simulink model "simulate_DSBSC"  (R2021a)
settings: Solver=VariableStepAuto  StartTime=0.0  StopTime=0.1  RelTol=1e-3
InitFcn:
  | fs = 4000;
  | frameSize = 1;
libraries: dspsrcs4 x4, commanapbnd3 x2, dsparch4 x1
settings Model: Creator=Byung-Jun Jang  LastModifiedBy=user
settings SolverCC: AlgebraicLoopSolver=TrustRegion
settings DataIOCC: ReturnWorkspaceOutputs=off
settings DebuggingCC: SFMachineParentedDataDiag=warning  ArithmeticOperatorsInVariantConditions=warning
settings SFSimCC: SimUseLocalCustomCode=off  CustomCodeUndefinedFunction=UseInterfaceOnly
settings RTWCC: RTWUseLocalCustomCode=off
settings CodeAppCC: StateflowObjectComments=on
settings SimscapeCC: SimscapeNormalizeSystem=off

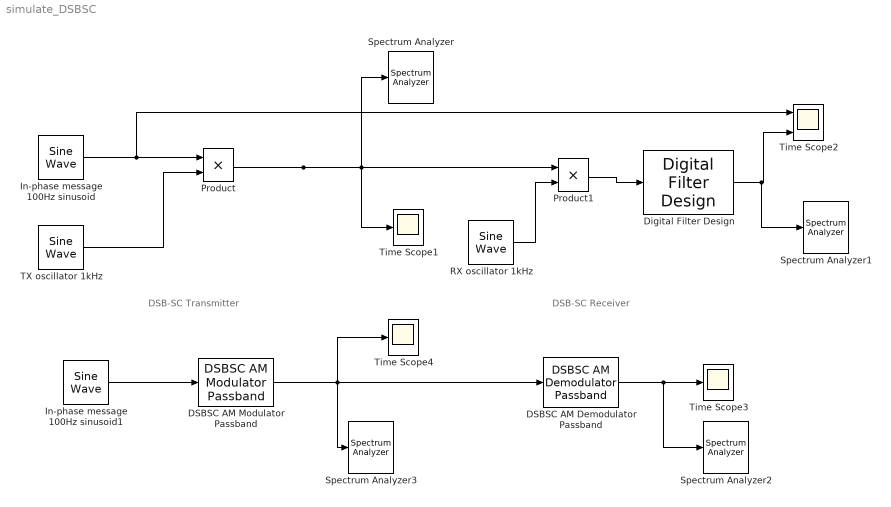
== system simulate_DSBSC ==
  note: DSB-SC Transmitter
  note: DSB-SC Receiver
  DSBSC AM Demodulator Passband : commanapbnd3/DSBSC AM Demodulator Passband  Fc=1000  Ph=0  method=Butterworth  n=4  cf=300  Rp=0.1  Rs=50
      settings: SourceProductBaseCode=CM
  DSBSC AM Modulator Passband : commanapbnd3/DSBSC AM Modulator Passband  Fc=1000  Ph=0
      settings: SourceProductBaseCode=CM
  Digital Filter Design : dsparch4/Digital Filter Design  mwdsp_browser_bugfix_var=off
  In-phase message 100Hz sinusoid : dspsrcs4/Sine Wave  Amplitude=1  Frequency=100  Phase=90  SampleMode=Discrete  OutComplex=Real  CompMethod=Trigonometric fcn  TableSize=Speed  SampleTime=1/fs  SamplesPerFrame=frameSize  ResetState=Restart at time zero  OutputFrames=off  dataType=double  wordLen=16  udDataType=sfix(16)  fracBitsMode=Best precision  numFracBits=15  OutDataTypeStr=double  LastOutDataTypeStr=double
  In-phase message 100Hz sinusoid1 : dspsrcs4/Sine Wave  Amplitude=1  Frequency=100  Phase=90  SampleMode=Discrete  OutComplex=Real  CompMethod=Trigonometric fcn  TableSize=Speed  SampleTime=1/fs  SamplesPerFrame=frameSize  ResetState=Restart at time zero  OutputFrames=off  dataType=double  wordLen=16  udDataType=sfix(16)  fracBitsMode=Best precision  numFracBits=15  OutDataTypeStr=double  LastOutDataTypeStr=double
  Product : Product
  Product1 : Product
  RX oscillator 1kHz : dspsrcs4/Sine Wave  Amplitude=1  Frequency=1000  Phase=0  SampleMode=Discrete  OutComplex=Real  CompMethod=Trigonometric fcn  TableSize=Speed  SampleTime=1/fs  SamplesPerFrame=frameSize  ResetState=Restart at time zero  OutputFrames=off  dataType=double  wordLen=16  udDataType=sfix(16)  fracBitsMode=Best precision  numFracBits=15  OutDataTypeStr=double  LastOutDataTypeStr=double
  Spectrum Analyzer{,1..3} (4 alike) : SpectrumAnalyzer
  TX oscillator 1kHz : dspsrcs4/Sine Wave  Amplitude=1  Frequency=1000  Phase=0  SampleMode=Discrete  OutComplex=Real  CompMethod=Trigonometric fcn  TableSize=Speed  SampleTime=1/fs  SamplesPerFrame=frameSize  ResetState=Restart at time zero  OutputFrames=off  dataType=double  wordLen=16  udDataType=sfix(16)  fracBitsMode=Best precision  numFracBits=15  OutDataTypeStr=double  LastOutDataTypeStr=double
  Time Scope1 : Scope
  Time Scope2 : Scope  NumInputPorts=2
  Time Scope3 : Scope
  Time Scope4 : Scope
  wires:
  In-phase message 100Hz sinusoid/1 -> Time Scope2/1, Product/1
  Product/1 -> Spectrum Analyzer/1, Product1/1, Time Scope1/1
  TX oscillator 1kHz/1 -> Product/2
  RX oscillator 1kHz/1 -> Product1/2
  Product1/1 -> Digital Filter Design/1
  Digital Filter Design/1 -> Spectrum Analyzer1/1, Time Scope2/2
  DSBSC AM Modulator Passband/1 -> Time Scope4/1, Spectrum Analyzer3/1, DSBSC AM Demodulator Passband/1
  In-phase message 100Hz sinusoid1/1 -> DSBSC AM Modulator Passband/1
  DSBSC AM Demodulator Passband/1 -> Spectrum Analyzer2/1, Time Scope3/1
